simulink model "operational_space_pd_w_g_comp"  (R2021b)
settings: Solver=VariableStepAuto  StartTime=0.0  StopTime=10.0  RelTol=1e-3
undefined symbols (not defined in the file): dqi, g_q, KD, KP, myRobot, qf, qi, xd
libraries: vrlib x1
settings Model: Creator=miche  LastModifiedBy=luigi

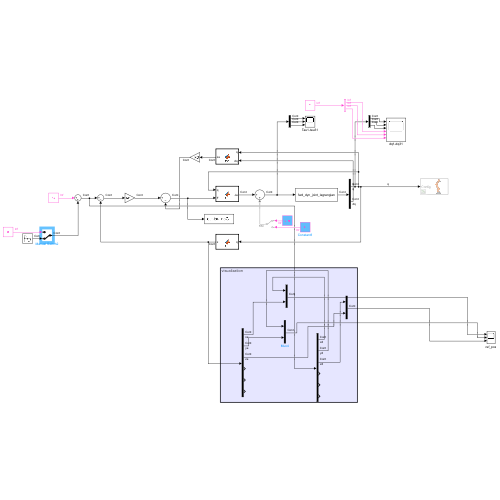
[thumbnail: Simulink's stored preview of the top-level diagram]
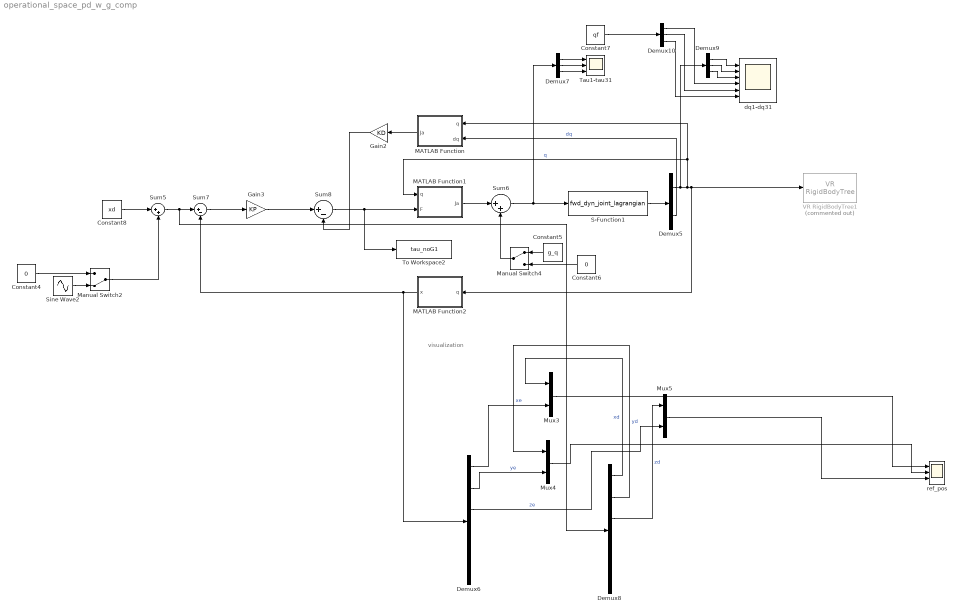
== system operational_space_pd_w_g_comp ==
  note: visualization
  Constant4 : Constant  Value=0
  Constant5 : Constant  Value=g_q
  Constant6 : Constant  Value=0
  Constant7 : Constant  Value=qf
  Constant8 : Constant  Value=xd
  Demux10 : Demux  Outputs=3
  Demux5 : Demux  Outputs=2
  Demux6 : Demux  Outputs=6
  Demux7 : Demux  Outputs=3
  Demux8 : Demux  Outputs=6
  Demux9 : Demux  Outputs=3
  Gain2 : Gain  Gain=KD
  Gain3 : Gain  Gain=KP
  MATLAB Function : MATLAB Function  TreatAsAtomicUnit=on
  MATLAB Function1 : MATLAB Function  TreatAsAtomicUnit=on
  MATLAB Function2 : MATLAB Function  TreatAsAtomicUnit=on
  Manual Switch2 : ManualSwitch  CurrentSetting=0
  Manual Switch4 : ManualSwitch
  Mux3 : Mux  Inputs=2
  Mux4 : Mux  Inputs=2
  Mux5 : Mux  Inputs=2
  S-Function1 : S-Function  FunctionName=fwd_dyn_joint_lagrangian  Parameters=myRobot,qi,dqi  SFunctionDeploymentMode=off  EnableBusSupport=off
  Sine Wave2 : Sin  Amplitude=0.1  SampleTime=0
  Sum5 : Sum  Inputs=|++
  Sum6 : Sum  Inputs=|++
  Sum7 : Sum  Inputs=|+-
  Sum8 : Sum  Inputs=|+-
  Tau1-tau31 : Scope  NumInputPorts=3
  To Workspace2 : ToWorkspace  VariableName=tau_noG1  SaveFormat=Timeseries  SampleTime=-1
  VR RigidBodyTree1 : vrlib/VR RigidBodyTree  Commented=on  RBT=rbt  useRBT=on  Ts=-1  ForceViewerOpen=on
      settings: SourceProductBaseCode=SL
  dq1-dq31 : Scope  NumInputPorts=6
  ref_pos : Scope  NumInputPorts=3
  wires:
  Constant6/1 -> Manual Switch4/2
  Gain2/1 -> Sum8/2
  Manual Switch2/1 -> Sum5/2
  MATLAB Function/1(Ja) -> Gain2/1
  Sum8/1 -> MATLAB Function1/2(F), To Workspace2/1
  Constant4/1 -> Manual Switch2/1
  Sum7/1 -> Gain3/1
  S-Function1/1 -> Demux5/1
  Demux5/2 -> MATLAB Function/2(dq)  "dq"
  Gain3/1 -> Sum8/1
  Sine Wave2/1 -> Manual Switch2/2
  Constant8/1 -> Sum5/1
  Constant5/1 -> Manual Switch4/1
  MATLAB Function1/1(Ja) -> Sum6/1
  Sum6/1 -> Demux7/1, S-Function1/1
  Demux7/3 -> Tau1-tau31/3
  Demux7/1 -> Tau1-tau31/1
  Demux7/2 -> Tau1-tau31/2
  Demux9/1 -> dq1-dq31/1
  Demux9/2 -> dq1-dq31/2
  Demux5/1 -> VR RigidBodyTree1/1, MATLAB Function2/1(q), MATLAB Function1/1(q), MATLAB Function/1(q), Demux9/1  "q"
  Demux9/3 -> dq1-dq31/3
  Manual Switch4/1 -> Sum6/2
  Demux10/1 -> dq1-dq31/4
  Demux10/2 -> dq1-dq31/5
  Demux10/3 -> dq1-dq31/6
  Constant7/1 -> Demux10/1
  Mux3/1 -> ref_pos/1
  Mux4/1 -> ref_pos/2
  Mux5/1 -> ref_pos/3
  Sum5/1 -> Demux8/1, Sum7/1
  MATLAB Function2/1(x) -> Demux6/1, Sum7/2
  Demux6/2 -> Mux4/2  "ye"
  Demux6/3 -> Mux5/2  "ze"
  Demux8/2 -> Mux4/1  "yd"
  Demux8/1 -> Mux3/1  "xd"
  Demux6/1 -> Mux3/2  "xe"
  Demux8/3 -> Mux5/1  "zd"

== matlab function operational_space_pd_w_g_comp/MATLAB Function1 ==
  data: q input size=3; Ja output size=3; F input
function Ja = fcn(q, F)

Ja = getJa(q)'*F;

== matlab function operational_space_pd_w_g_comp/MATLAB Function2 ==
  data: q input; x output
function x = fcn(q)
x = getK(q);

== matlab function operational_space_pd_w_g_comp/MATLAB Function ==
  data: q input size=3; Ja output; dq input
function Ja = fcn(q, dq)

Ja = getJa(q)*dq;
